simulink model "EMFwithData"  (Simulink 7.4)
settings: Solver=ode45  StartTime=0.0  StopTime=10.0  RelTol=1e-3
settings Model: Creator=dread  LastModifiedBy=dread

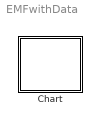
== system EMFwithData ==
  Chart : Stateflow chart

== matlab function Chart ==
  data: in1 function_input double; in2 function_input double; out1 function_output double; out2 function_output double; const constant double size=1; local local double size=[1,2]; const constant double; localVar local double
function [out1, out2] = emf(in1, in2)
out1 = in2;
out2 = in1;
